simulink model "HW7_PartA"  (R2025b)
settings: Solver=ode45  StartTime=0.0  StopTime=3  MaxStep=0.005  RelTol=1e-6
settings Model: Creator=dixiao  LastModifiedBy=dixiao

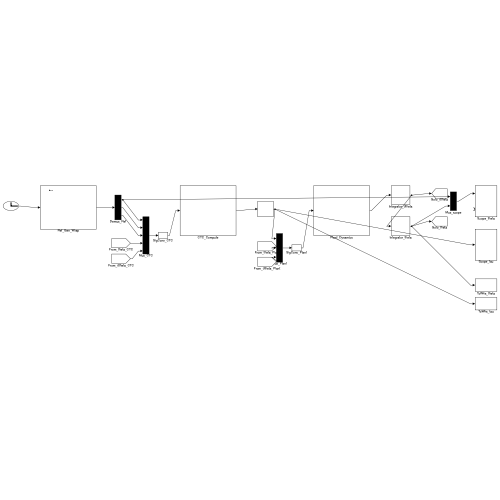
[thumbnail: Simulink's stored preview of the top-level diagram]
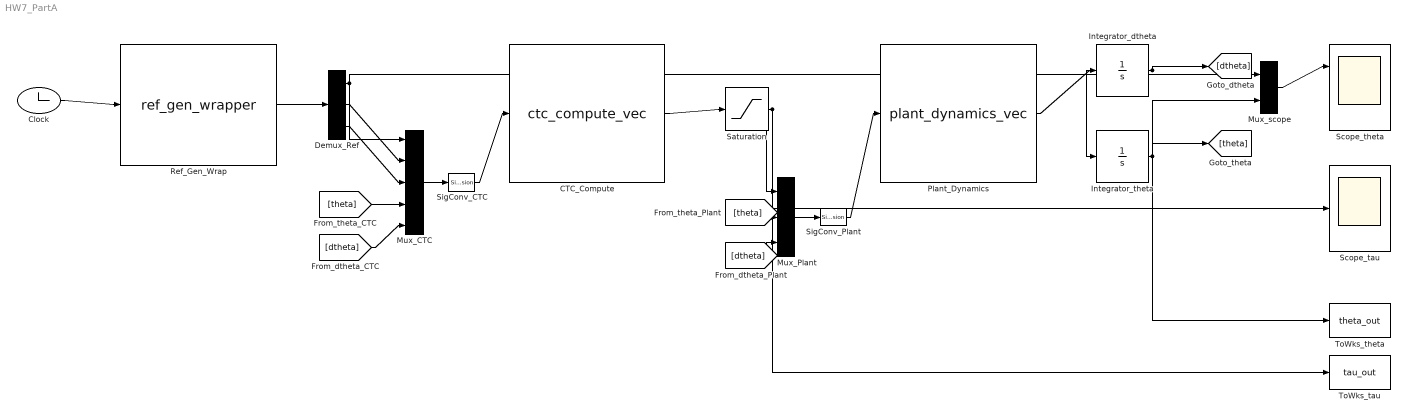
== system HW7_PartA ==
  CTC_Compute : MATLABFcn  MATLABFcn=ctc_compute_vec  OutputDimensions=4
  Clock : Clock
  Demux_Ref : Demux  Outputs=[4 4 4]
  Integrator_dtheta : Integrator  InitialCondition=[0; 0; 0; 0]
  Integrator_theta : Integrator  InitialCondition=[0.3*pi; 0.2*pi; 0.35*pi; -0.03]
  Mux_CTC : Mux  Inputs=5
  Mux_Plant : Mux  Inputs=3
  Mux_scope : Mux  Inputs=2
  Plant_Dynamics : MATLABFcn  MATLABFcn=plant_dynamics_vec  OutputDimensions=4
  Ref_Gen_Wrap : MATLABFcn  MATLABFcn=ref_gen_wrapper  OutputDimensions=12
  Saturation : Saturate  UpperLimit=[6000; 2000; 1000; 100]  LowerLimit=[-6000; -2000; -1000; -100]
  Scope_tau : Scope
  Scope_theta : Scope  NumInputPorts=2
  SigConv_CTC : SignalConversion  OverrideOpt=off
  SigConv_Plant : SignalConversion  OverrideOpt=off
  ToWks_tau : ToWorkspace  VariableName=tau_out  SampleTime=-1
  ToWks_theta : ToWorkspace  VariableName=theta_out  SampleTime=-1
  wires:
  Clock/1 -> Ref_Gen_Wrap/1
  Ref_Gen_Wrap/1 -> Demux_Ref/1
  Demux_Ref/1 -> Mux_CTC/1, Mux_scope/1
  Demux_Ref/2 -> Mux_CTC/2
  Demux_Ref/3 -> Mux_CTC/3
  [theta] -> Mux_CTC/4
  [dtheta] -> Mux_CTC/5
  Mux_CTC/1 -> SigConv_CTC/1
  SigConv_CTC/1 -> CTC_Compute/1
  CTC_Compute/1 -> Saturation/1
  Saturation/1 -> Mux_Plant/1, Scope_tau/1, ToWks_tau/1
  [theta] -> Mux_Plant/2
  [dtheta] -> Mux_Plant/3
  Mux_Plant/1 -> SigConv_Plant/1
  SigConv_Plant/1 -> Plant_Dynamics/1
  Plant_Dynamics/1 -> Integrator_dtheta/1
  Integrator_dtheta/1 -> Integrator_theta/1, [dtheta]
  Integrator_theta/1 -> [theta], Mux_scope/2, ToWks_theta/1
  Mux_scope/1 -> Scope_theta/1
